simulink model "Ornek3_11"  (R2021b)
settings: Solver=VariableStepAuto  StartTime=0.0  StopTime=10.0  RelTol=1e-3
libraries: commsrccod2 x2, dspvision x1
settings Model: Creator=MONSTER  LastModifiedBy=MONSTER

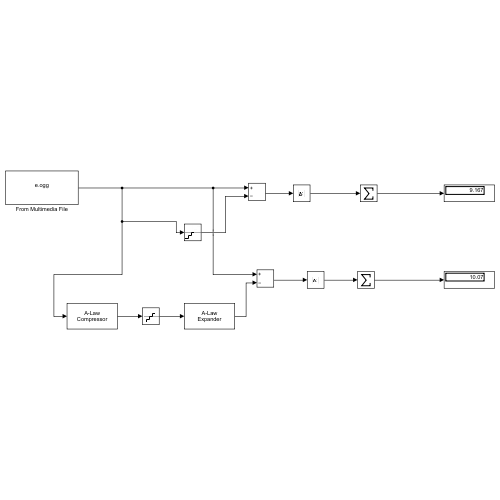
[thumbnail: Simulink's stored preview of the top-level diagram]
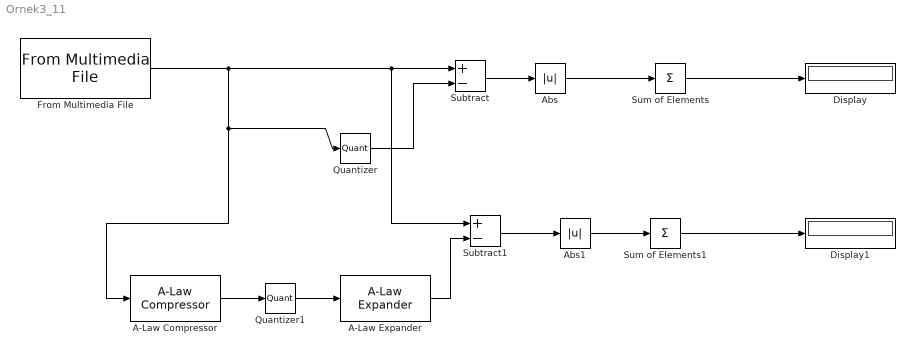
== system Ornek3_11 ==
  A-Law Compressor : commsrccod2/A-Law Compressor  A=87.6  V=1
      settings: SourceProductBaseCode=CM
  A-Law Expander : commsrccod2/A-Law Expander  A=87.6  V=1
      settings: SourceProductBaseCode=CM
  Abs : Abs
  Abs1 : Abs
  Display : Display
  Display1 : Display
  From Multimedia File : dspvision/From Multimedia File  inputFilename=C:\Users\MONSTER\OneDrive\Belgeler\e.ogg  readRange=[1 Inf]  loop=on  numPlays=inf  outputStreams=Audio only  videoDataType=single  audioDataType=double  inheritSampleTime=on  userDefinedSampleTime=1/30  noAudioOutput=off  isIntensityVideo=off  fourcc=RGB  colorVideoFormat=Separate color signals  outputEOF=off  dataOrg=Column-major  audioFrameSize=1024  computeAudioFrameSize=off  outSamplingMode=Sample based
  Quantizer : Quantizer
  Quantizer1 : Quantizer
  Subtract : Sum  Inputs=+-
  Subtract1 : Sum  Inputs=+-
  Sum of Elements : Sum  Inputs=+
  Sum of Elements1 : Sum  Inputs=+
  wires:
  Quantizer/1 -> Subtract/2
  Subtract/1 -> Abs/1
  Abs/1 -> Sum of Elements/1
  Sum of Elements/1 -> Display/1
  Subtract1/1 -> Abs1/1
  Abs1/1 -> Sum of Elements1/1
  Sum of Elements1/1 -> Display1/1
  A-Law Expander/1 -> Subtract1/2
  Quantizer1/1 -> A-Law Expander/1
  A-Law Compressor/1 -> Quantizer1/1
  From Multimedia File/1 -> Subtract1/1, Subtract/1, Quantizer/1, A-Law Compressor/1
